simulink subsystem "Bluetooth_Umbrales"  (R2024b)
settings: Solver=VariableStepAuto  StartTime=0.0  StopTime=10.0  RelTol=1e-3
settings Model: Creator=Chenfu  LastModifiedBy=Chenfu

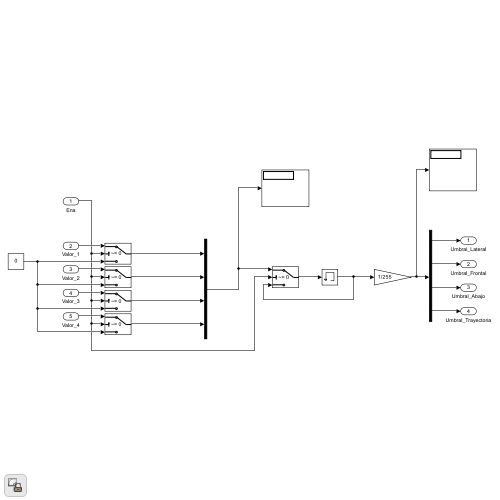
[thumbnail: Simulink's stored preview of the top-level diagram]
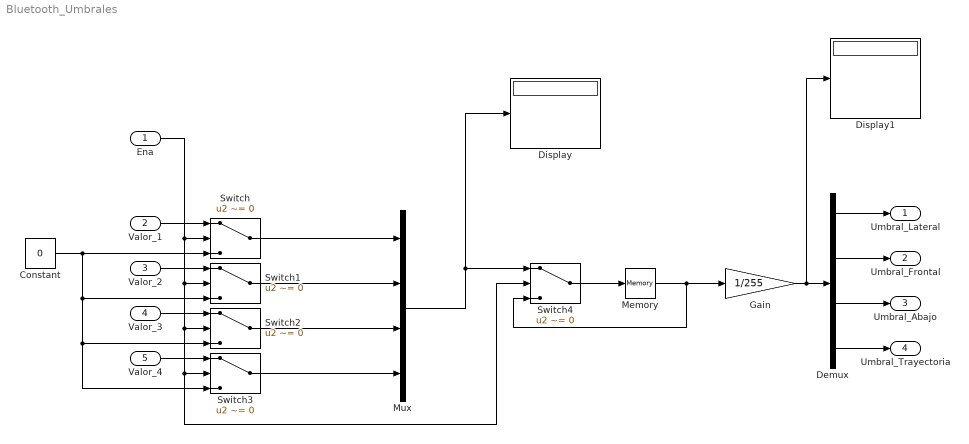
== system Bluetooth_Umbrales ==
  Ena : Inport
  Valor_1 : Inport  Port=2
  Valor_2 : Inport  Port=3
  Valor_3 : Inport  Port=4
  Valor_4 : Inport  Port=5
  Constant : Constant  Value=0  OutDataTypeStr='uint8'
  Demux : Demux
  Display : Display
  Display1 : Display
  Gain : Gain  Gain=1/255  OutDataTypeStr='double'
  Memory : Memory  InitialCondition=25
  Mux : Mux
  Switch{,1..4} (5 alike) : Switch  Criteria=u2 ~= 0  SaturateOnIntegerOverflow=off  InputSameDT=off
  Umbral_Lateral : Outport
  Umbral_Frontal : Outport  Port=2
  Umbral_Abajo : Outport  Port=3
  Umbral_Trayectoria : Outport  Port=4
  wires:
  Switch3/1 -> Mux/4
  Valor_4/1 -> Switch3/1
  Valor_3/1 -> Switch2/1
  Valor_2/1 -> Switch1/1
  Constant/1 -> Switch1/3, Switch3/3, Switch2/3, Switch/3
  Ena/1 -> Switch/2, Switch1/2, Switch4/2, Switch3/2, Switch2/2
  Valor_1/1 -> Switch/1
  Memory/1 -> Switch4/3, Gain/1
  Switch1/1 -> Mux/2
  Switch/1 -> Mux/1
  Switch2/1 -> Mux/3
  Demux/1 -> Umbral_Lateral/1
  Demux/2 -> Umbral_Frontal/1
  Demux/3 -> Umbral_Abajo/1
  Switch4/1 -> Memory/1
  Mux/1 -> Switch4/1, Display/1
  Gain/1 -> Demux/1, Display1/1
  Demux/4 -> Umbral_Trayectoria/1
